simulink model "FindMinOfTwoSig_WithoutMinBlk"  (R2018b)
settings: Solver=VariableStepAuto  StartTime=0.0  StopTime=10.0  RelTol=1e-3
libraries: standard_autocodable_blockset x2
settings Model: Creator=SKHOT2  LastModifiedBy=SKHOT2

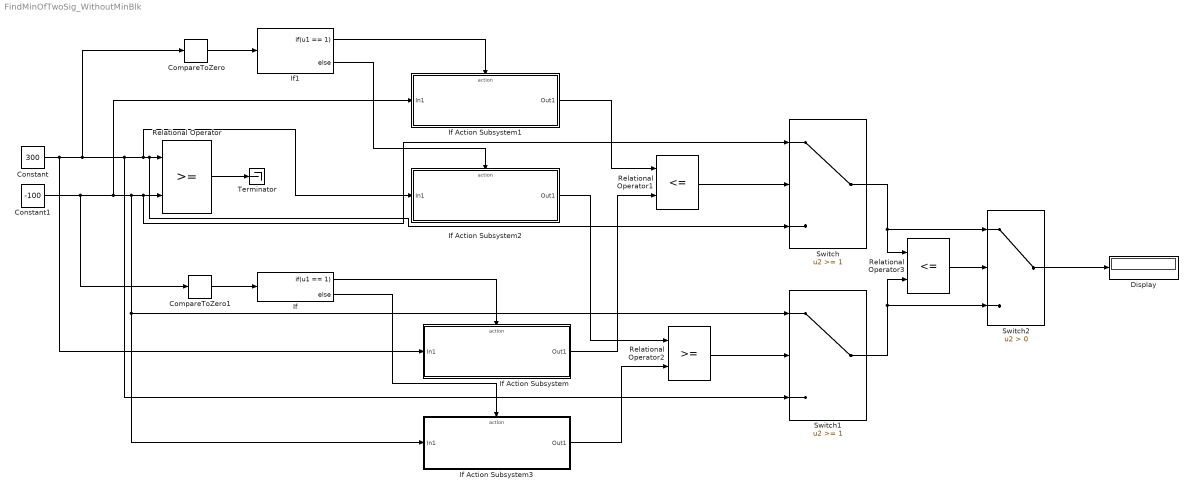
== system FindMinOfTwoSig_WithoutMinBlk ==
  CompareToZero : standard_autocodable_blockset/Logic and Bit Operations/CompareToZero  relop=<=  OutDataTypeStr=boolean  ZeroCross=off
      settings: SourceProductName=Ford Standard Autocodable Blockset
  CompareToZero1 : standard_autocodable_blockset/Logic and Bit Operations/CompareToZero  relop=<=  OutDataTypeStr=boolean  ZeroCross=off
      settings: SourceProductName=Ford Standard Autocodable Blockset
  Constant : Constant  Value=300
  Constant1 : Constant  Value=-100
  Display : Display
  If : If  IfExpression=u1 == 1
  If Action Subsystem : Subsystem  TreatAsAtomicUnit=on
  If Action Subsystem1 : Subsystem  TreatAsAtomicUnit=on
  If Action Subsystem2 : Subsystem  TreatAsAtomicUnit=on
  If Action Subsystem3 : Subsystem  TreatAsAtomicUnit=on
  If1 : If  IfExpression=u1 == 1
  Relational Operator : RelationalOperator  OutDataTypeStr=boolean  RndMeth=Simplest
  Relational Operator1 : RelationalOperator  Operator=<=  OutDataTypeStr=boolean  RndMeth=Simplest
  Relational Operator2 : RelationalOperator  OutDataTypeStr=boolean  RndMeth=Simplest
  Relational Operator3 : RelationalOperator  Operator=<=  OutDataTypeStr=boolean  RndMeth=Simplest
  Switch : Switch  Threshold=1
  Switch1 : Switch  Threshold=1
  Switch2 : Switch  Criteria=u2 > Threshold
  Terminator : Terminator
  wires:
  Constant1/1 -> CompareToZero1/1, If Action Subsystem1/1(In1), Switch1/1, If Action Subsystem3/1(In1), Switch/1, Relational Operator/2
  Constant/1 -> If Action Subsystem/1(In1), CompareToZero/1, Switch1/3, If Action Subsystem2/1(In1), Switch/3, Relational Operator/1
  CompareToZero1/1 -> If/1
  If/1 -> If Action Subsystem/Action
  CompareToZero/1 -> If1/1
  If1/1 -> If Action Subsystem1/Action
  If1/2 -> If Action Subsystem2/Action
  If/2 -> If Action Subsystem3/Action
  If Action Subsystem1/1(Out1) -> Relational Operator1/1
  If Action Subsystem/1(Out1) -> Relational Operator1/2
  If Action Subsystem2/1(Out1) -> Relational Operator2/1
  If Action Subsystem3/1(Out1) -> Relational Operator2/2
  Relational Operator1/1 -> Switch/2
  Relational Operator2/1 -> Switch1/2
  Switch1/1 -> Relational Operator3/2, Switch2/3
  Relational Operator3/1 -> Switch2/2
  Switch2/1 -> Display/1
  Switch/1 -> Switch2/1, Relational Operator3/1
  Relational Operator/1 -> Terminator/1

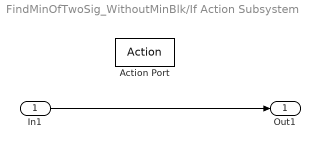
== system FindMinOfTwoSig_WithoutMinBlk/If Action Subsystem ==
  In1 : Inport
  Action Port : ActionPort  ActionType=then
  Out1 : Outport
  wires:
  In1/1 -> Out1/1

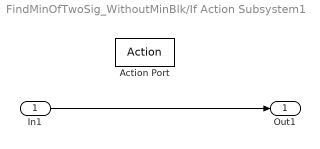
== system FindMinOfTwoSig_WithoutMinBlk/If Action Subsystem1 ==
  In1 : Inport
  Action Port : ActionPort  ActionType=then
  Out1 : Outport
  wires:
  In1/1 -> Out1/1

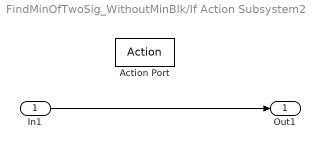
== system FindMinOfTwoSig_WithoutMinBlk/If Action Subsystem2 ==
  In1 : Inport
  Action Port : ActionPort  ActionType=else
  Out1 : Outport
  wires:
  In1/1 -> Out1/1

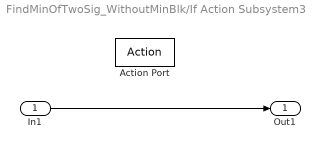
== system FindMinOfTwoSig_WithoutMinBlk/If Action Subsystem3 ==
  In1 : Inport
  Action Port : ActionPort  ActionType=else
  Out1 : Outport
  wires:
  In1/1 -> Out1/1
